simulink model "OrientationTestAnimation"  (R2022b)
settings: Solver=VariableStepAuto  StartTime=0.0  StopTime=100  RelTol=1e-3
libraries: vrlib x1
settings Model: Creator=jjwan  LastModifiedBy=jjwan

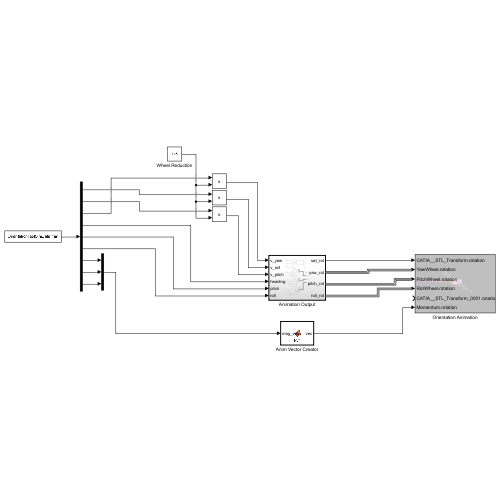
[thumbnail: Simulink's stored preview of the top-level diagram]
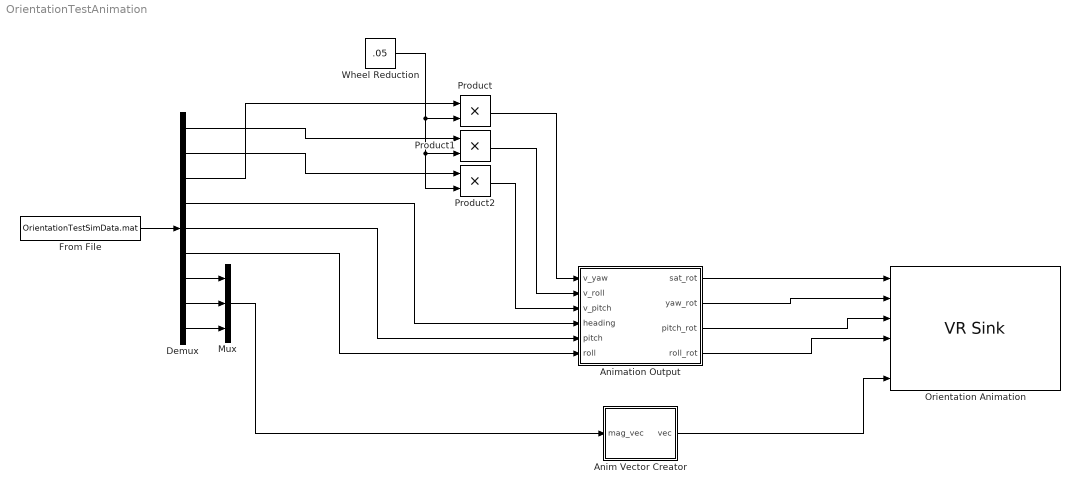
== system OrientationTestAnimation ==
  Anim Vector Creator : MATLAB Function  TreatAsAtomicUnit=on
  Animation Output : Subsystem  TreatAsAtomicUnit=on
  Demux : Demux  Outputs=9
  From File : FromFile  FileName=OrientationTestSimData.mat  SampleTime=0
  Mux : Mux  Inputs=3
  Orientation Animation : vrlib/VR Sink  InstantiateOnLoad=on  SampleTime=.02  ViewEnable=on  RemoteChange=off  RemoteView=off  FieldsWritten=CATIA__STL_Transform.rotation.4.1.1.double#YawWheel.rotation.4.1.1.double#PitchWheel.rotation.4.1.1.double#RollWheel.rotation.4.1.1.double#CATIA__STL_Transform_0001.rotation.4.1.1.double#Momentum.rotation.4.1.1.double  WorldFileName=SatVR.x3d  AutoView=off  VideoDimensions=[]  AllowVariableSize=off  FigureProperties="{'Position', 'Name', 'Viewpoint', 'CameraBound', 'CameraDirection', 'CameraPosition', 'CameraUpVector', 'ZoomFactor', 'Antialiasing', 'Headlight', 'Lighting', 'NavPanel', 'Sound', 'StatusBar', 'Stereo3D', 'Stereo3DCameraOffset', 'Stereo3DHIT', 'ToolBar', 'Textures', 'Transparency', 'Triad', 'Wireframe', 'NavZones', 'NavMode', 'NavSpeed', 'CaptureFileFormat', 'CaptureFileName', 'Record2DCompressMethod', 'Record2DCompressQuality', 'Record2D', 'Record2DFileName', 'Record2DFPS'; [1.0000000000000000e+00  -1.0058000000000002e+03   1.9200000000000000e+03   9.0680000000000018e+02], '', '', 'on', [7.4676088066681012e-01  -6.6501230007218681e-01  -1.0335756309539590e-02], [-1.0419430785644620e+03   9.4664764342009858e+02  -2.2512815203859873e+01], [-6.5450491128537736e-02  -8.8943330452295674e-02   9.9388395558994247e-01], [1.0000000000000000e+00], 'on', 'on', 'on', 'halfbar', 'on', 'on', 'off', [1.0000000149011612e-01], [0.0000000000000000e+00], 'on', 'on', 'on', 'none', 'off', 'off', 'examine', 'normal', 'png', '%f_anim_%n.png', 'auto', [1.0000000000000000e+02], 'on', '%f_anim_%n.avi', 'auto'}"
  Product : Product
  Product1 : Product
  Product2 : Product
  Wheel Reduction : Constant  Value=.05
  wires:
  Animation Output/1(sat_rot) -> Orientation Animation/1
  Animation Output/2(yaw_rot) -> Orientation Animation/2
  Animation Output/4(roll_rot) -> Orientation Animation/4
  Animation Output/3(pitch_rot) -> Orientation Animation/3
  Anim Vector Creator/1(vec) -> Orientation Animation/6
  Product2/1 -> Animation Output/3(v_pitch)
  Wheel Reduction/1 -> Product2/2, Product1/2, Product/2
  Product1/1 -> Animation Output/2(v_roll)
  Product/1 -> Animation Output/1(v_yaw)
  From File/1 -> Demux/1
  Mux/1 -> Anim Vector Creator/1(mag_vec)
  Demux/7 -> Mux/1
  Demux/8 -> Mux/2
  Demux/9 -> Mux/3
  Demux/6 -> Animation Output/6(roll)
  Demux/5 -> Animation Output/5(pitch)
  Demux/4 -> Animation Output/4(heading)
  Demux/1 -> Product1/1
  Demux/2 -> Product2/1
  Demux/3 -> Product/1

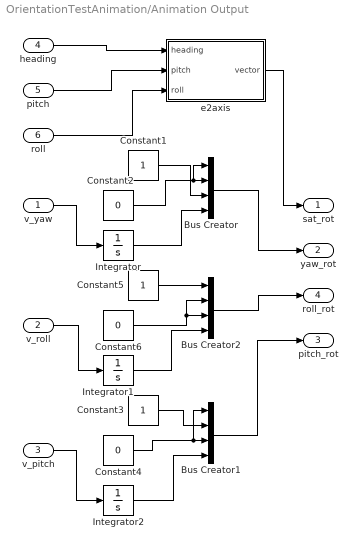
== system OrientationTestAnimation/Animation Output ==
  v_yaw : Inport
  v_roll : Inport  Port=2
  v_pitch : Inport  Port=3
  heading : Inport  Port=4
  pitch : Inport  Port=5
  roll : Inport  Port=6
  Bus Creator : BusCreator  Inputs=4
  Bus Creator1 : BusCreator  Inputs=4
  Bus Creator2 : BusCreator  Inputs=4
  Constant1 : Constant
  Constant2 : Constant  Value=0
  Constant3 : Constant
  Constant4 : Constant  Value=0
  Constant5 : Constant
  Constant6 : Constant  Value=0
  Integrator : Integrator
  Integrator1 : Integrator
  Integrator2 : Integrator
  e2axis : MATLAB Function  TreatAsAtomicUnit=on
  sat_rot : Outport
  yaw_rot : Outport  Port=2
  pitch_rot : Outport  Port=3
  roll_rot : Outport  Port=4
  wires:
  Constant6/1 -> Bus Creator2/2, Bus Creator2/3
  Constant5/1 -> Bus Creator2/1
  Constant1/1 -> Bus Creator/3
  Constant3/1 -> Bus Creator1/2
  Constant2/1 -> Bus Creator/1, Bus Creator/2
  Constant4/1 -> Bus Creator1/1, Bus Creator1/3
  heading/1 -> e2axis/1(heading)
  pitch/1 -> e2axis/2(pitch)
  roll/1 -> e2axis/3(roll)
  e2axis/1(vector) -> sat_rot/1
  v_yaw/1 -> Integrator/1
  v_roll/1 -> Integrator1/1
  v_pitch/1 -> Integrator2/1
  Bus Creator/1 -> yaw_rot/1
  Bus Creator2/1 -> roll_rot/1
  Bus Creator1/1 -> pitch_rot/1
  Integrator/1 -> Bus Creator/4
  Integrator1/1 -> Bus Creator2/4
  Integrator2/1 -> Bus Creator1/4

== matlab function OrientationTestAnimation/Animation Output/e2axis ==
  data: heading input; pitch input; roll input; vector output

function vector = e2axis(heading, pitch, roll)

% eul = [heading -pitch roll];
% coder.extrinsic('eul2rotm');
% coder.extrinsic('rotm2axang');
% rotm = eul2rotm(eul,'ZYX');
% v = rotm2axang(rotm);
% vector = [0;0;0;0];
% vector(1) = v(1);
% vector(2) = v(2);
% vector(3) = v(3);
% vector(4) = v(4);

% converts Tait-Bryan angles to quaternion
    cy = cos(heading/2);    sy = sin(heading/2);    % Trig yaw terms
    cp = cos(pitch/2);  sp = sin(pitch/2);  % Trig pitch terms
    cr = cos(roll/2);    sr = sin(roll/2);    % Trig roll terms

    q = [cr*cp*cy + sr*sp*sy;
         sr*cp*cy - cr*sp*sy;
         cr*sp*cy + sr*cp*sy;
         cr*cp*sy - sr*sp*cy];

    angle = 2*atan2(norm(q(2:4)),q(1));
    axis = q(2:4)/sin(angle/2);
    vector = [axis(1); axis(2); axis(3); angle];
end

== matlab function OrientationTestAnimation/Anim Vector Creator ==
  data: mag_vec input; vec output
function vec = fcn(mag_vec)

if norm(mag_vec) < 10^-10
    mag_vec = [0;0;0];
end

if norm(mag_vec) == 0
    theta = 0;
else
    cos_theta = mag_vec(3) / sqrt(mag_vec(1)^2+mag_vec(2)^2+mag_vec(3)^2);
    theta = acos(cos_theta);
end
    
vec = [-mag_vec(2); mag_vec(1); 0; theta];
